simulink model "HeatExchange"  (R2025a)
settings: Solver=VariableStepAuto  StartTime=0.0  StopTime=500  RelTol=1e-3
libraries: nesl_utility x27, SimscapeFluids_lib x13, fl_lib x8
settings Model: Creator=20112  LastModifiedBy=20112
settings DataIOCC: SignalLogging=off
settings DebuggingCC: ReadBeforeWriteMsg=DisableAll  WriteAfterWriteMsg=DisableAll  WriteAfterReadMsg=DisableAll  MultiTaskDSMMsg=none
settings ModelReferenceCC: UpdateModelReferenceTargets=IfOutOfDate
settings SFSimCC: SFSimEcho=off
settings SimscapeCC: SimscapeLogType=all  SimscapeCompileComponentReuse=on  SimscapeCompileArtifactsDiskCache=on

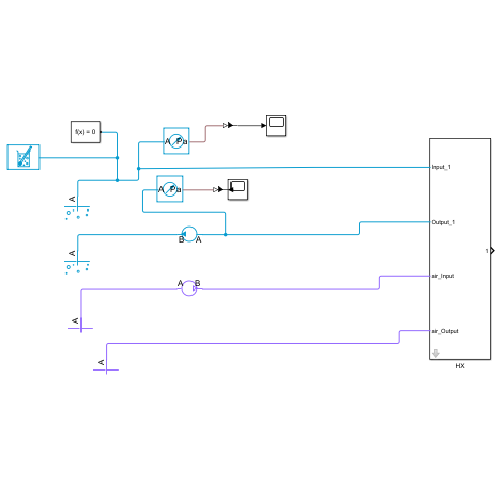
[thumbnail: Simulink's stored preview of the top-level diagram]
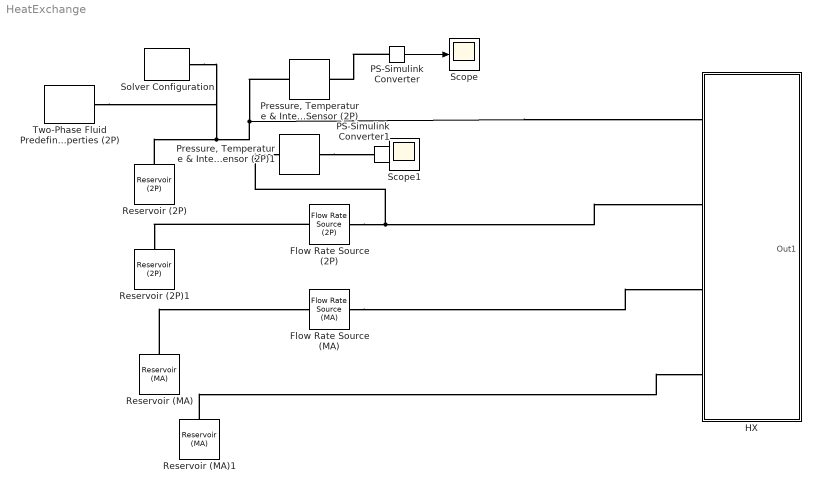
== system HeatExchange ==
  Flow Rate Source (2P) : fl_lib/Two-Phase Fluid/Sources/Flow Rate Source (2P)  source_type=foundation.enum.constant_controlled.constant  flow_type=foundation.enum.mass_volumetric_flow.mass  mass_flow=3e-3 kg/s  volumetric_flow=0 m^3/s  power_spec=foundation.enum.power_spec.none  area_A=pi*(5e-3)^2/4 m^2  area_B=pi*(5e-3)^2/4 m^2
      settings: InternalSimscapePortConfiguration="{\"Bottom\":[],\"Left\":[{\"id\":\"A\",\"label\":\"A\",\"type\":\"foundation.two_phase_fluid.two_phase_fluid\"}],\"Right\":[{\"id\":\"B\",\"label\":\"B\",\"type\":\"foundation.two_phase_fluid.two_phase_fluid\"}],\"Top\":[]}"
  Flow Rate Source (MA) : fl_lib/Moist Air/Sources/Flow Rate Source (MA)  source_type=foundation.enum.constant_controlled.constant  flow_type=foundation.enum.mass_volumetric_flow.mass  mass_flow=2 kg/s  volumetric_flow=0 m^3/s  volumetric_flow_conditions=foundation.enum.volumetric_flow_conditions.actual  p_std=0.101325 MPa  T_std=20 degC  RH_std=0.65  power_spec=foundation.enum.power_spec.none  area_A=1*1*0.7 m^2  area_B=1*1*0.7 m^2
      settings: InternalSimscapePortConfiguration="{\"Bottom\":[],\"Left\":[{\"id\":\"A\",\"label\":\"A\",\"type\":\"foundation.moist_air.moist_air\"}],\"Right\":[{\"id\":\"B\",\"label\":\"B\",\"type\":\"foundation.moist_air.moist_air\"}],\"Top\":[]}"
  HX : Subsystem  mask{Cross_sectional_area_A1=pi*(5e-3)^2/4, Cross_sectional_area_B1=pi*(5e-3)^2/4, Cross_sectional_area_A2=1*1*0.7, Cross_sectional_area_B2=1*1*0.7, Total_length_each_tube=1, Tube_inner_diameter=5e-3, Agg_equiv_length=0.03, Internal_surface_roughness=15e-6, Initial_pressure=2.5, Initial_temperature=323, Length_tube_segment=1, Tube_outer_diameter=6e-3, Longitudinal_tube_pitch=0.15, Transverse_tube_pitch=0.15, Fouling_factor_air=0.1, Total_fin_surface_area_air=0, Fin_efficiency_air=0.5, Initial_pressure_air=0.101325, Initial_temperature_air=293.15, Initial_rel_humidity=0.5}
      mask prompts: Cross_sectional_area_A1 "Cross-sectional area at port A1 (m²):"; Cross_sectional_area_B1 "Cross-sectional area at port B1 (m²):"; Cross_sectional_area_A2 "Cross-sectional area at port A2 (m²):"; Cross_sectional_area_B2 "Cross-sectional area at port B2 (m²):"; Total_length_each_tube "Total length of each tube (m):"; Tube_inner_diameter "Tube inner diameter (m):"; Agg_equiv_length "Aggregate equivalent length of local resistances (m):"; Internal_surface_roughness "Internal surface absolute roughness (m):"; Initial_pressure "Initial two-phase fluid pressure (MPa):"; Initial_temperature "Initial two-phase fluid temperature (K):"; Length_tube_segment "Length of each tube segment in row (m):"; Tube_outer_diameter "Tube outer diameter (m):"; Longitudinal_tube_pitch "Longitudinal tube pitch (along flow direction) (m):"; Transverse_tube_pitch "Transverse tube pitch (perpendicular to flow) (m):"; Fouling_factor_air "Fouling factor (K*m²/kW):"; Total_fin_surface_area_air "Total fin surface area (m²):"; Fin_efficiency_air "Fin efficiency:"; Initial_pressure_air "Initial moist air pressure (MPa):"; Initial_temperature_air "Initial moist air temperature (K):"; Initial_rel_humidity "Initial moist air relative humidity:"
  PS-Simulink Converter : nesl_utility/PS-Simulink Converter  PhysicalDomain=network_engine_domain  SubClassName=ps_output  LeftPortType=input  RightPortType=output  PseudoPeriodic=off  Frequencies=[]  VectorFormat=inherit  Unit=inherit  AffineConversion=off
  PS-Simulink Converter1 : nesl_utility/PS-Simulink Converter  PhysicalDomain=network_engine_domain  SubClassName=ps_output  LeftPortType=input  RightPortType=output  PseudoPeriodic=off  Frequencies=[]  VectorFormat=inherit  Unit=inherit  AffineConversion=off
  "Pressure, Temperature & Internal Energy Sensor (2P)" : fl_lib/Two-Phase Fluid/Sensors/Pressure, Temperature & Internal Energy Sensor (2P)  reference=foundation.enum.MeasurementReference.absolute  pressure=true  pressure_spec=foundation.enum.PressureMeasementSpec.Absolute  temperature=false  internal_energy=false
      settings: InternalSimscapePortConfiguration="{\"Bottom\":[],\"Left\":[{\"id\":\"A\",\"label\":\"A\",\"type\":\"foundation.two_phase_fluid.two_phase_fluid\"}],\"Right\":[{\"id\":\"Pa\",\"label\":\"Pa\",\"type\":\"output\"}],\"Top\":[]}"
  "Pressure, Temperature & Internal Energy Sensor (2P)1" : fl_lib/Two-Phase Fluid/Sensors/Pressure, Temperature & Internal Energy Sensor (2P)  reference=foundation.enum.MeasurementReference.absolute  pressure=true  pressure_spec=foundation.enum.PressureMeasementSpec.Absolute  temperature=false  internal_energy=false
      settings: InternalSimscapePortConfiguration="{\"Bottom\":[],\"Left\":[{\"id\":\"A\",\"label\":\"A\",\"type\":\"foundation.two_phase_fluid.two_phase_fluid\"}],\"Right\":[{\"id\":\"Pa\",\"label\":\"Pa\",\"type\":\"output\"}],\"Top\":[]}"
  Reservoir (2P) : fl_lib/Two-Phase Fluid/Elements/Reservoir (2P)  pressure_spec=foundation.enum.ReservoirPressureSpec2P.Specified  reservoir_pressure=2.5 MPa  reservoir_condensing_temperature=373.15 K  reservoir_evaporating_temperature=373.15 K  energy_spec=foundation.enum.ReservoirEnergySpec2P.Temperature  reservoir_temperature=323 K  reservoir_quality=0.5  reservoir_void_fraction=0.5  reservoir_enthalpy=1500 kJ/kg  reservoir_internal_energy=1500 kJ/kg  reservoir_subcooling=5 deltaK  reservoir_superheating=5 deltaK  area_A=pi*(5e-3)^2/4 m^2
  Reservoir (2P)1 : fl_lib/Two-Phase Fluid/Elements/Reservoir (2P)  pressure_spec=foundation.enum.ReservoirPressureSpec2P.Specified  reservoir_pressure=2.5 MPa  reservoir_condensing_temperature=373.15 K  reservoir_evaporating_temperature=373.15 K  energy_spec=foundation.enum.ReservoirEnergySpec2P.Temperature  reservoir_temperature=300 K  reservoir_quality=0.5  reservoir_void_fraction=0.5  reservoir_enthalpy=1500 kJ/kg  reservoir_internal_energy=1500 kJ/kg  reservoir_subcooling=5 deltaK  reservoir_superheating=5 deltaK  area_A=pi*(5e-3)^2/4 m^2
  Reservoir (MA) : fl_lib/Moist Air/Elements/Reservoir (MA)  pressure_input=false  pressure_spec=foundation.enum.pressure_spec.atmospheric  reservoir_pressure=0.101325 MPa  temperature_input=false  temperature_spec=foundation.enum.temperature_spec.atmospheric  reservoir_temperature=293.15 K  humidity_input=false  humidity_spec=foundation.enum.HumiditySpec.RelativeHumidity  reservoir_RH=0.5  reservoir_x_w=0.01  reservoir_y_w=0.01  reservoir_HR=0.01  reservoir_Tw=287 K  trace_gas_input=false  trace_gas_spec=foundation.enum.trace_gas_spec.mass_fraction  reservoir_x_g=0.001  reservoir_y_g=0.001  water_droplets_input=false  reservoir_r_d=0  RH_ws=1  area_A=1*1*0.7 m^2  input_error_spec=foundation.enum.input_range_error.warn
  Reservoir (MA)1 : fl_lib/Moist Air/Elements/Reservoir (MA)  pressure_input=false  pressure_spec=foundation.enum.pressure_spec.atmospheric  reservoir_pressure=0.101325 MPa  temperature_input=false  temperature_spec=foundation.enum.temperature_spec.atmospheric  reservoir_temperature=293.15 K  humidity_input=false  humidity_spec=foundation.enum.HumiditySpec.RelativeHumidity  reservoir_RH=0.5  reservoir_x_w=0.01  reservoir_y_w=0.01  reservoir_HR=0.01  reservoir_Tw=287 K  trace_gas_input=false  trace_gas_spec=foundation.enum.trace_gas_spec.mass_fraction  reservoir_x_g=0.001  reservoir_y_g=0.001  water_droplets_input=false  reservoir_r_d=0  RH_ws=1  area_A=1*1*0.7 m^2  input_error_spec=foundation.enum.input_range_error.warn
  Scope : Scope
      settings: ActiveDisplayYMinimum=2.4952076318398331  ActiveDisplayYMaximum=2.506118752797994
  Scope1 : Scope
      settings: ActiveDisplayYMinimum=2.4945864565577294  ActiveDisplayYMaximum=2.495223080796356
  Solver Configuration : nesl_utility/Solver Configuration  PhysicalDomain=network_engine_domain  SubClassName=solver  LeftPortType=input  RightPortType=generic  Tones=[]  Harmonics=[]  SimulateNoise=off  Profile=off  UseLocalSampling=off  EnableSwitchedLinearOptims=on  FrequencyDomain=off  UseCCode=off  RelTol=0.001  AbsTol=0.001  MinStep=1e-09  ToWorkspace=off  RevertToSquareIcSolve=off  NumHomotopyIterations=100  PhasorMode=off  PhasorModeNumHarmonics=1  ConsistencySolver=NEWTON_XTOL_AFTER_FTOL  IndexReductionMethod=DerivativeReplacement  DoDC=off  ResidualTolerance=1e-09  ConsistencyTolSource=GLOBAL  ConsistencyAbsTol=0.001  ConsistencyRelTol=0.001  ConsistencyTolFactor=0.001  UseLocalSolver=off  LocalSolverChoice=NE_BACKWARD_EULER_ADVANCER  ResolveIndetEquations=on  FunctionEvalNumThread=1  LocalSolverSampleTime=0.001  DoFixedCost=off  MaxNonlinIter=3  MaxModeIter=2  ComputeImpulses=off  ImpulseIterations=2  LinearAlgebra=auto  LinearAlgebraNumThread=0  EquationFormulation=NE_TIME_EF  DelaysMemoryBudget=1024  AutomaticFiltering=on  FilteringTimeConstant=0.001  PartitionStorageMethod=AS_NEEDED  PartitionMemoryBudget=1024  PartitionMethod=ROBUST  MultibodyUseLocalSolver=off  MultibodyLocalSolverChoice=ODE1  MultibodyLocalSolverSampleTime=0.001
  Two-Phase Fluid Predefined Properties (2P) : SimscapeFluids_lib/Two-Phase Fluid/Utilities/Two-Phase Fluid Predefined Properties (2P)  fluid=fluids.two_phase_fluid.utilities.enum.Fluid.R32  p_atm=0.101325 MPa  properties_range_check=simscape.enum.assert.action.error  q_rev=0.01 Pa
  wires:
  PS-Simulink Converter/1 -> Scope/1
  PS-Simulink Converter1/1 -> Scope1/1
  connections:
  Reservoir (2P)/LConn1 -- Two-Phase Fluid Predefined Properties (2P)/RConn1 -- Solver Configuration/RConn1 -- "Pressure, Temperature & Internal Energy Sensor (2P)"/LConn1 -- HX/LConn1
  Flow Rate Source (2P)/RConn1 -- Reservoir (2P)1/LConn1
  Flow Rate Source (2P)/LConn1 -- "Pressure, Temperature & Internal Energy Sensor (2P)1"/LConn1 -- HX/LConn2
  Reservoir (MA)/LConn1 -- Flow Rate Source (MA)/LConn1
  Flow Rate Source (MA)/RConn1 -- HX/LConn3
  Reservoir (MA)1/LConn1 -- HX/LConn4
  PS-Simulink Converter/LConn1 -- "Pressure, Temperature & Internal Energy Sensor (2P)"/RConn1
  "Pressure, Temperature & Internal Energy Sensor (2P)1"/RConn1 -- PS-Simulink Converter1/LConn1

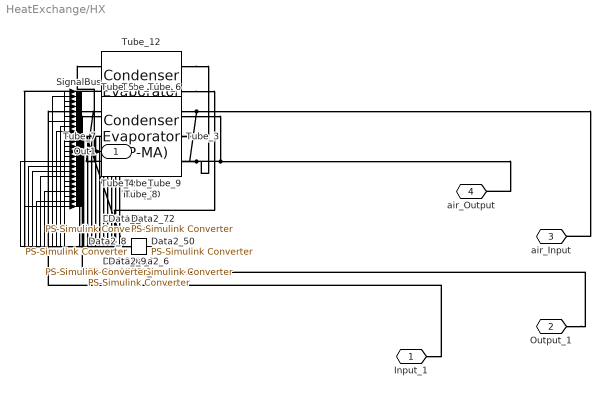
== system HeatExchange/HX ==
  Data1_{1..12} (12 alike) : nesl_utility/PS-Simulink Converter  PhysicalDomain=network_engine_domain  SubClassName=ps_output  LeftPortType=input  RightPortType=output  PseudoPeriodic=off  Frequencies=[]  VectorFormat=inherit  Unit=inherit  AffineConversion=off
  Data2_{1..12} (12 alike) : nesl_utility/PS-Simulink Converter  PhysicalDomain=network_engine_domain  SubClassName=ps_output  LeftPortType=input  RightPortType=output  PseudoPeriodic=off  Frequencies=[]  VectorFormat=inherit  Unit=inherit  AffineConversion=off
  SignalBus : BusCreator  Inputs=24
  Tube_1 : SimscapeFluids_lib/Heat Exchangers/Two-Phase Fluid - Moist Air/Condenser Evaporator (2P-MA)  flow_arrangement=fluids.heat_exchangers.enum.FlowArrangement2PMA.Cross  cross_flow_arrangement=fluids.heat_exchangers.enum.CrossFlowArrangement2PMA.UnmixedUnmixed  R_wall=1000*log(Tube_outer_diameter/Tube_inner_diameter)/(2*pi*Length_tube_segment*380) K/kW  wall_thermal_mass=false  mass_wall=1 kg  cp_wall=490 J/(K*kg)  area_A1=Cross_sectional_area_A1 m^2  area_B1=pi*Tube_inner_diameter^2/4 m^2  area_A2=Cross_sectional_area_A2/4 m^2  area_B2=Cross_sectional_area_B2/4 m^2  tube_num_2P=1  tube_length_2P=Total_length_each_tube m  tube_cross_section_2P=fluids.heat_exchangers.enum.TubeCrossSection.Circular  tube_diameter_2P=Tube_inner_diameter m  tube_width_2P=0.05 m  tube_height_2P=0.05 m  tube_inner_diameter_2P=0.05 m  tube_outer_diameter_2P=0.1 m  tube_flow_area_2P=0.002 m^2  tube_wetted_perimeter_2P=0.15 m  tube_heat_perimeter_2P=0.15 m  tube_pressure_loss_spec_2P=fluids.heat_exchangers.enum.TubePressureLossSpec2P.Haaland  tube_loss_coeff_2P=10  tube_local_pressure_loss_spec_2P=fluids.heat_exchangers.enum.LocalLossSpec.AggregateLength  tube_length_add_2P=Agg_equiv_length m  tube_local_loss_coefficient_2P=0.1  tube_roughness_pressure_2P=Internal_surface_roughness m  tube_Re_lam_pressure_2P=2000  tube_Re_tur_pressure_2P=4000  tube_shape_factor_generic_2P=64  tube_heat_coeff_spec_2P=fluids.heat_exchangers.enum.TubeHeatCoeffSpec2P.GneilinskiCavalliniZecchin  tube_colburn_coeff_liq_2P=[.023, .8, .33]  tube_colburn_coeff_mix_2P=[.05, .8, .33]  tube_colburn_coeff_vap_2P=[.023, .8, .33]  tube_roughness_heat_2P=15e-6 m  tube_Re_lam_heat_2P=2000  tube_Re_tur_heat_2P=4000  tube_Nu_lam_generic_2P=3.66  fouling_factor_2P=0.1 K*m^2/kW  fin_area_2P=0 m^2  fin_efficiency_2P=0.5  energy_spec_2P=foundation.enum.energy_spec.temperature  p_init_2P=Initial_pressure MPa  T_init_2P=Initial_temperature K  x_init_2P=0.5  alpha_init_2P=0.5  h_init_2P=1500 kJ/kg  u_init_2P=1500 kJ/kg  flow_geometry_MA=fluids.heat_exchangers.enum.FlowGeometryMA.AcrossTubeBank  tube_num_MA=25  tube_length_MA=1 m  tube_cross_section_MA=fluids.heat_exchangers.enum.TubeCrossSection.Circular  tube_diameter_MA=0.05 m  tube_width_MA=0.05 m  tube_height_MA=0.05 m  tube_inner_diameter_MA=0.05 m  tube_outer_diameter_MA=0.1 m  tube_flow_area_MA=0.002 m^2  tube_wetted_perimeter_MA=0.15 m  tube_heat_perimeter_MA=0.15 m  tube_pressure_loss_spec_MA=fluids.heat_exchangers.enum.TubePressureLossSpec.Haaland  tube_loss_coeff_MA=10  tube_local_pressure_loss_spec_MA=fluids.heat_exchangers.enum.LocalLossSpec.AggregateLength  tube_length_add_MA=0.1 m  tube_local_loss_coefficient_MA=0.1  tube_roughness_pressure_MA=15e-6 m  tube_Re_lam_pressure_MA=2000  tube_Re_tur_pressure_MA=4000  tube_shape_factor_generic_MA=64  tube_heat_coeff_spec_MA=fluids.heat_exchangers.enum.TubeHeatCoeffSpec.Gneilinski  tube_colburn_coeff_MA=[.023, .8, .33]  tube_roughness_heat_MA=15e-6 m  tube_Re_lam_heat_MA=2000  tube_Re_tur_heat_MA=4000  tube_Nu_lam_generic_MA=3.66  bank_arrangement_MA=fluids.heat_exchangers.enum.BankArrangement.Inline  bank_num_rows_MA=1  bank_tubes_per_row_MA=1  bank_width_MA=Length_tube_segment m  bank_tube_diameter_MA=Tube_outer_diameter m  bank_longitudinal_pitch_MA=Longitudinal_tube_pitch m  bank_transverse_pitch_MA=Transverse_tube_pitch m  bank_pressure_loss_spec_MA=fluids.heat_exchangers.enum.BankPressureLossSpec.Martin  bank_euler_MA=10  bank_heat_coeff_spec_MA=fluids.heat_exchangers.enum.BankHeatCoeffSpec.Martin  bank_colburn_coeff_MA=[.27, .63, .36]  generic_flow_area_MA=0.01 m^2  generic_heat_area_MA=2 m^2  generic_volume_MA=0.05 m^3  generic_loss_coeff_MA=10  generic_colburn_coeff_MA=[.023, .8, .33]  fouling_factor_MA=Fouling_factor_air K*m^2/kW  fin_area_MA=Total_fin_surface_area_air m^2  fin_efficiency_MA=Fin_efficiency_air  p_init_MA=Initial_pressure_air MPa  T_init_MA=Initial_temperature_air K  humidity_spec_MA=foundation.enum.HumiditySpec.RelativeHumidity  RH_init_MA=Initial_rel_humidity  x_w_init_MA=0.01  y_w_init_MA=0.01  HR_init_MA=0.01  Tw_init_MA=287 K  trace_gas_spec_MA=foundation.enum.trace_gas_spec.mass_fraction  x_g_init_MA=0.001  y_g_init_MA=0.001  r_d_init_MA=0  RH_ws_MA=1  time_constant_cond_MA=1e-3 s  time_constant_evap_MA=1e-3 s  fraction_entrained_MA=1
      settings: InternalSimscapePortConfiguration="{\"Bottom\":[],\"Left\":[{\"id\":\"A1\",\"label\":\"A1\",\"type\":\"foundation.two_phase_fluid.two_phase_fluid\"},{\"id\":\"Z\",\"label\":\"Z\",\"type\":\"output\"},{\"id\":\"B1\",\"label\":\"B1\",\"type\":\"foundation.two_phase_fluid.two_phase_fluid\"}],\"Right\":[{\"id\":\"A2\",\"label\":\"A2\",\"type\":\"foundation.moist_air.moist_air\"},{\"id\":\"W\",\"label\":\"W\",\"type\":\"output\"},{\"id\":\"B2\",\"label\":\"B2\",\"type\":\"foundation.moist_air.moist_air\"}],\"Top\":[]}"
  Tube_{2..11} (10 alike) : SimscapeFluids_lib/Heat Exchangers/Two-Phase Fluid - Moist Air/Condenser Evaporator (2P-MA)  flow_arrangement=fluids.heat_exchangers.enum.FlowArrangement2PMA.Cross  cross_flow_arrangement=fluids.heat_exchangers.enum.CrossFlowArrangement2PMA.UnmixedUnmixed  R_wall=1000*log(Tube_outer_diameter/Tube_inner_diameter)/(2*pi*Length_tube_segment*380) K/kW  wall_thermal_mass=false  mass_wall=1 kg  cp_wall=490 J/(K*kg)  area_A1=pi*Tube_inner_diameter^2/4 m^2  area_B1=pi*Tube_inner_diameter^2/4 m^2  area_A2=Cross_sectional_area_A2/4 m^2  area_B2=Cross_sectional_area_B2/4 m^2  tube_num_2P=1  tube_length_2P=Total_length_each_tube m  tube_cross_section_2P=fluids.heat_exchangers.enum.TubeCrossSection.Circular  tube_diameter_2P=Tube_inner_diameter m  tube_width_2P=0.05 m  tube_height_2P=0.05 m  tube_inner_diameter_2P=0.05 m  tube_outer_diameter_2P=0.1 m  tube_flow_area_2P=0.002 m^2  tube_wetted_perimeter_2P=0.15 m  tube_heat_perimeter_2P=0.15 m  tube_pressure_loss_spec_2P=fluids.heat_exchangers.enum.TubePressureLossSpec2P.Haaland  tube_loss_coeff_2P=10  tube_local_pressure_loss_spec_2P=fluids.heat_exchangers.enum.LocalLossSpec.AggregateLength  tube_length_add_2P=Agg_equiv_length m  tube_local_loss_coefficient_2P=0.1  tube_roughness_pressure_2P=Internal_surface_roughness m  tube_Re_lam_pressure_2P=2000  tube_Re_tur_pressure_2P=4000  tube_shape_factor_generic_2P=64  tube_heat_coeff_spec_2P=fluids.heat_exchangers.enum.TubeHeatCoeffSpec2P.GneilinskiCavalliniZecchin  tube_colburn_coeff_liq_2P=[.023, .8, .33]  tube_colburn_coeff_mix_2P=[.05, .8, .33]  tube_colburn_coeff_vap_2P=[.023, .8, .33]  tube_roughness_heat_2P=15e-6 m  tube_Re_lam_heat_2P=2000  tube_Re_tur_heat_2P=4000  tube_Nu_lam_generic_2P=3.66  fouling_factor_2P=0.1 K*m^2/kW  fin_area_2P=0 m^2  fin_efficiency_2P=0.5  energy_spec_2P=foundation.enum.energy_spec.temperature  p_init_2P=Initial_pressure MPa  T_init_2P=Initial_temperature K  x_init_2P=0.5  alpha_init_2P=0.5  h_init_2P=1500 kJ/kg  u_init_2P=1500 kJ/kg  flow_geometry_MA=fluids.heat_exchangers.enum.FlowGeometryMA.AcrossTubeBank  tube_num_MA=25  tube_length_MA=1 m  tube_cross_section_MA=fluids.heat_exchangers.enum.TubeCrossSection.Circular  tube_diameter_MA=0.05 m  tube_width_MA=0.05 m  tube_height_MA=0.05 m  tube_inner_diameter_MA=0.05 m  tube_outer_diameter_MA=0.1 m  tube_flow_area_MA=0.002 m^2  tube_wetted_perimeter_MA=0.15 m  tube_heat_perimeter_MA=0.15 m  tube_pressure_loss_spec_MA=fluids.heat_exchangers.enum.TubePressureLossSpec.Haaland  tube_loss_coeff_MA=10  tube_local_pressure_loss_spec_MA=fluids.heat_exchangers.enum.LocalLossSpec.AggregateLength  tube_length_add_MA=0.1 m  tube_local_loss_coefficient_MA=0.1  tube_roughness_pressure_MA=15e-6 m  tube_Re_lam_pressure_MA=2000  tube_Re_tur_pressure_MA=4000  tube_shape_factor_generic_MA=64  tube_heat_coeff_spec_MA=fluids.heat_exchangers.enum.TubeHeatCoeffSpec.Gneilinski  tube_colburn_coeff_MA=[.023, .8, .33]  tube_roughness_heat_MA=15e-6 m  tube_Re_lam_heat_MA=2000  tube_Re_tur_heat_MA=4000  tube_Nu_lam_generic_MA=3.66  bank_arrangement_MA=fluids.heat_exchangers.enum.BankArrangement.Inline  bank_num_rows_MA=1  bank_tubes_per_row_MA=1  bank_width_MA=Length_tube_segment m  bank_tube_diameter_MA=Tube_outer_diameter m  bank_longitudinal_pitch_MA=Longitudinal_tube_pitch m  bank_transverse_pitch_MA=Transverse_tube_pitch m  bank_pressure_loss_spec_MA=fluids.heat_exchangers.enum.BankPressureLossSpec.Martin  bank_euler_MA=10  bank_heat_coeff_spec_MA=fluids.heat_exchangers.enum.BankHeatCoeffSpec.Martin  bank_colburn_coeff_MA=[.27, .63, .36]  generic_flow_area_MA=0.01 m^2  generic_heat_area_MA=2 m^2  generic_volume_MA=0.05 m^3  generic_loss_coeff_MA=10  generic_colburn_coeff_MA=[.023, .8, .33]  fouling_factor_MA=Fouling_factor_air K*m^2/kW  fin_area_MA=Total_fin_surface_area_air m^2  fin_efficiency_MA=Fin_efficiency_air  p_init_MA=Initial_pressure_air MPa  T_init_MA=Initial_temperature_air K  humidity_spec_MA=foundation.enum.HumiditySpec.RelativeHumidity  RH_init_MA=Initial_rel_humidity  x_w_init_MA=0.01  y_w_init_MA=0.01  HR_init_MA=0.01  Tw_init_MA=287 K  trace_gas_spec_MA=foundation.enum.trace_gas_spec.mass_fraction  x_g_init_MA=0.001  y_g_init_MA=0.001  r_d_init_MA=0  RH_ws_MA=1  time_constant_cond_MA=1e-3 s  time_constant_evap_MA=1e-3 s  fraction_entrained_MA=1
      settings: InternalSimscapePortConfiguration="{\"Bottom\":[],\"Left\":[{\"id\":\"A1\",\"label\":\"A1\",\"type\":\"foundation.two_phase_fluid.two_phase_fluid\"},{\"id\":\"Z\",\"label\":\"Z\",\"type\":\"output\"},{\"id\":\"B1\",\"label\":\"B1\",\"type\":\"foundation.two_phase_fluid.two_phase_fluid\"}],\"Right\":[{\"id\":\"A2\",\"label\":\"A2\",\"type\":\"foundation.moist_air.moist_air\"},{\"id\":\"W\",\"label\":\"W\",\"type\":\"output\"},{\"id\":\"B2\",\"label\":\"B2\",\"type\":\"foundation.moist_air.moist_air\"}],\"Top\":[]}"
  Tube_12 : SimscapeFluids_lib/Heat Exchangers/Two-Phase Fluid - Moist Air/Condenser Evaporator (2P-MA)  flow_arrangement=fluids.heat_exchangers.enum.FlowArrangement2PMA.Cross  cross_flow_arrangement=fluids.heat_exchangers.enum.CrossFlowArrangement2PMA.UnmixedUnmixed  R_wall=1000*log(Tube_outer_diameter/Tube_inner_diameter)/(2*pi*Length_tube_segment*380) K/kW  wall_thermal_mass=false  mass_wall=1 kg  cp_wall=490 J/(K*kg)  area_A1=pi*Tube_inner_diameter^2/4 m^2  area_B1=Cross_sectional_area_B1 m^2  area_A2=Cross_sectional_area_A2/4 m^2  area_B2=Cross_sectional_area_B2/4 m^2  tube_num_2P=1  tube_length_2P=Total_length_each_tube m  tube_cross_section_2P=fluids.heat_exchangers.enum.TubeCrossSection.Circular  tube_diameter_2P=Tube_inner_diameter m  tube_width_2P=0.05 m  tube_height_2P=0.05 m  tube_inner_diameter_2P=0.05 m  tube_outer_diameter_2P=0.1 m  tube_flow_area_2P=0.002 m^2  tube_wetted_perimeter_2P=0.15 m  tube_heat_perimeter_2P=0.15 m  tube_pressure_loss_spec_2P=fluids.heat_exchangers.enum.TubePressureLossSpec2P.Haaland  tube_loss_coeff_2P=10  tube_local_pressure_loss_spec_2P=fluids.heat_exchangers.enum.LocalLossSpec.AggregateLength  tube_length_add_2P=Agg_equiv_length m  tube_local_loss_coefficient_2P=0.1  tube_roughness_pressure_2P=Internal_surface_roughness m  tube_Re_lam_pressure_2P=2000  tube_Re_tur_pressure_2P=4000  tube_shape_factor_generic_2P=64  tube_heat_coeff_spec_2P=fluids.heat_exchangers.enum.TubeHeatCoeffSpec2P.GneilinskiCavalliniZecchin  tube_colburn_coeff_liq_2P=[.023, .8, .33]  tube_colburn_coeff_mix_2P=[.05, .8, .33]  tube_colburn_coeff_vap_2P=[.023, .8, .33]  tube_roughness_heat_2P=15e-6 m  tube_Re_lam_heat_2P=2000  tube_Re_tur_heat_2P=4000  tube_Nu_lam_generic_2P=3.66  fouling_factor_2P=0.1 K*m^2/kW  fin_area_2P=0 m^2  fin_efficiency_2P=0.5  energy_spec_2P=foundation.enum.energy_spec.temperature  p_init_2P=Initial_pressure MPa  T_init_2P=Initial_temperature K  x_init_2P=0.5  alpha_init_2P=0.5  h_init_2P=1500 kJ/kg  u_init_2P=1500 kJ/kg  flow_geometry_MA=fluids.heat_exchangers.enum.FlowGeometryMA.AcrossTubeBank  tube_num_MA=25  tube_length_MA=1 m  tube_cross_section_MA=fluids.heat_exchangers.enum.TubeCrossSection.Circular  tube_diameter_MA=0.05 m  tube_width_MA=0.05 m  tube_height_MA=0.05 m  tube_inner_diameter_MA=0.05 m  tube_outer_diameter_MA=0.1 m  tube_flow_area_MA=0.002 m^2  tube_wetted_perimeter_MA=0.15 m  tube_heat_perimeter_MA=0.15 m  tube_pressure_loss_spec_MA=fluids.heat_exchangers.enum.TubePressureLossSpec.Haaland  tube_loss_coeff_MA=10  tube_local_pressure_loss_spec_MA=fluids.heat_exchangers.enum.LocalLossSpec.AggregateLength  tube_length_add_MA=0.1 m  tube_local_loss_coefficient_MA=0.1  tube_roughness_pressure_MA=15e-6 m  tube_Re_lam_pressure_MA=2000  tube_Re_tur_pressure_MA=4000  tube_shape_factor_generic_MA=64  tube_heat_coeff_spec_MA=fluids.heat_exchangers.enum.TubeHeatCoeffSpec.Gneilinski  tube_colburn_coeff_MA=[.023, .8, .33]  tube_roughness_heat_MA=15e-6 m  tube_Re_lam_heat_MA=2000  tube_Re_tur_heat_MA=4000  tube_Nu_lam_generic_MA=3.66  bank_arrangement_MA=fluids.heat_exchangers.enum.BankArrangement.Inline  bank_num_rows_MA=1  bank_tubes_per_row_MA=1  bank_width_MA=Length_tube_segment m  bank_tube_diameter_MA=Tube_outer_diameter m  bank_longitudinal_pitch_MA=Longitudinal_tube_pitch m  bank_transverse_pitch_MA=Transverse_tube_pitch m  bank_pressure_loss_spec_MA=fluids.heat_exchangers.enum.BankPressureLossSpec.Martin  bank_euler_MA=10  bank_heat_coeff_spec_MA=fluids.heat_exchangers.enum.BankHeatCoeffSpec.Martin  bank_colburn_coeff_MA=[.27, .63, .36]  generic_flow_area_MA=0.01 m^2  generic_heat_area_MA=2 m^2  generic_volume_MA=0.05 m^3  generic_loss_coeff_MA=10  generic_colburn_coeff_MA=[.023, .8, .33]  fouling_factor_MA=Fouling_factor_air K*m^2/kW  fin_area_MA=Total_fin_surface_area_air m^2  fin_efficiency_MA=Fin_efficiency_air  p_init_MA=Initial_pressure_air MPa  T_init_MA=Initial_temperature_air K  humidity_spec_MA=foundation.enum.HumiditySpec.RelativeHumidity  RH_init_MA=Initial_rel_humidity  x_w_init_MA=0.01  y_w_init_MA=0.01  HR_init_MA=0.01  Tw_init_MA=287 K  trace_gas_spec_MA=foundation.enum.trace_gas_spec.mass_fraction  x_g_init_MA=0.001  y_g_init_MA=0.001  r_d_init_MA=0  RH_ws_MA=1  time_constant_cond_MA=1e-3 s  time_constant_evap_MA=1e-3 s  fraction_entrained_MA=1
      settings: InternalSimscapePortConfiguration="{\"Bottom\":[],\"Left\":[{\"id\":\"A1\",\"label\":\"A1\",\"type\":\"foundation.two_phase_fluid.two_phase_fluid\"},{\"id\":\"Z\",\"label\":\"Z\",\"type\":\"output\"},{\"id\":\"B1\",\"label\":\"B1\",\"type\":\"foundation.two_phase_fluid.two_phase_fluid\"}],\"Right\":[{\"id\":\"A2\",\"label\":\"A2\",\"type\":\"foundation.moist_air.moist_air\"},{\"id\":\"W\",\"label\":\"W\",\"type\":\"output\"},{\"id\":\"B2\",\"label\":\"B2\",\"type\":\"foundation.moist_air.moist_air\"}],\"Top\":[]}"
  Input_1 : PMIOPort  Side=Left
  Output_1 : PMIOPort  Port=2  Side=Left
  air_Input : PMIOPort  Port=3  Side=Left
  air_Output : PMIOPort  Port=4  Side=Left
  Out1 : Outport
  wires:
  Data1_7/1 -> SignalBus/13
  Data2_4/1 -> SignalBus/8
  Data1_5/1 -> SignalBus/9
  Data2_1/1 -> SignalBus/2
  Data1_4/1 -> SignalBus/7
  Data1_11/1 -> SignalBus/21
  Data2_9/1 -> SignalBus/18
  Data1_12/1 -> SignalBus/23
  Data1_9/1 -> SignalBus/17
  Data2_8/1 -> SignalBus/16
  Data2_12/1 -> SignalBus/24
  Data1_8/1 -> SignalBus/15
  Data1_1/1 -> SignalBus/1
  Data1_2/1 -> SignalBus/3
  Data2_5/1 -> SignalBus/10
  Data2_11/1 -> SignalBus/22
  Data1_3/1 -> SignalBus/5
  Data2_7/1 -> SignalBus/14
  Data2_3/1 -> SignalBus/6
  Data1_6/1 -> SignalBus/11
  Data2_6/1 -> SignalBus/12
  Data2_10/1 -> SignalBus/20
  Data1_10/1 -> SignalBus/19
  Data2_2/1 -> SignalBus/4
  SignalBus/1 -> Out1/1
  connections:
  Tube_10/LConn3 -- Tube_11/LConn1
  Tube_3/RConn3 -- Tube_12/RConn3 -- air_Output/RConn1 -- Tube_9/RConn3 -- Tube_6/RConn3
  Tube_9/LConn2 -- Data1_9/LConn1
  Tube_1/LConn2 -- Data1_1/LConn1
  Input_1/RConn1 -- Tube_1/LConn1
  Tube_9/RConn2 -- Data2_9/LConn1
  Tube_7/LConn3 -- Tube_10/LConn1
  Tube_6/LConn2 -- Data1_6/LConn1
  Tube_4/RConn2 -- Data2_4/LConn1
  Tube_9/RConn1 -- Tube_8/RConn3
  Tube_8/LConn2 -- Data1_8/LConn1
  Tube_4/LConn2 -- Data1_4/LConn1
  Tube_1/LConn3 -- Tube_4/LConn1
  Tube_12/LConn2 -- Data1_12/LConn1
  Tube_8/RConn2 -- Data2_8/LConn1
  Tube_5/LConn3 -- Tube_2/LConn1
  Tube_2/LConn3 -- Tube_3/LConn1
  Tube_1/RConn2 -- Data2_1/LConn1
  Tube_5/RConn2 -- Data2_5/LConn1
  Tube_1/RConn1 -- air_Input/RConn1 -- Tube_10/RConn1 -- Tube_7/RConn1 -- Tube_4/RConn1
  Tube_5/LConn2 -- Data1_5/LConn1
  Tube_3/LConn2 -- Data1_3/LConn1
  Tube_12/RConn2 -- Data2_12/LConn1
  Tube_10/LConn2 -- Data1_10/LConn1
  Tube_2/RConn2 -- Data2_2/LConn1
  Tube_11/RConn2 -- Data2_11/LConn1
  Tube_11/LConn2 -- Data1_11/LConn1
  Tube_6/RConn2 -- Data2_6/LConn1
  Tube_9/LConn3 -- Tube_12/LConn1
  Tube_3/RConn2 -- Data2_3/LConn1
  Tube_7/LConn2 -- Data1_7/LConn1
  Tube_7/RConn2 -- Data2_7/LConn1
  Tube_10/RConn2 -- Data2_10/LConn1
  Tube_2/LConn2 -- Data1_2/LConn1
  Tube_11/LConn3 -- Tube_8/LConn1
  Output_1/RConn1 -- Tube_12/LConn3
  Tube_4/LConn3 -- Tube_7/LConn1
  Tube_3/LConn3 -- Tube_6/LConn1
  Tube_8/LConn3 -- Tube_5/LConn1
  Tube_6/LConn3 -- Tube_9/LConn1
  Tube_5/RConn1 -- Tube_4/RConn3
  Tube_12/RConn1 -- Tube_11/RConn3
  Tube_8/RConn1 -- Tube_7/RConn3
  Tube_11/RConn1 -- Tube_10/RConn3
  Tube_6/RConn1 -- Tube_5/RConn3
  Tube_3/RConn1 -- Tube_2/RConn3
  Tube_2/RConn1 -- Tube_1/RConn3
